simulink model "pendule_simple"  (R2016a)
settings: Solver=VariableStepAuto  StartTime=0.0  StopTime=10.0  RelTol=1e-3
undefined symbols (not defined in the file): K
libraries: simulink x1
settings Model: Creator=tmeunier  LastModifiedBy=tmeunier

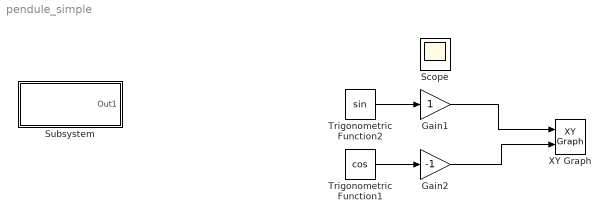
== system pendule_simple ==
  Gain1 : Gain
  Gain2 : Gain  Gain=-1
  Scope : Scope
  Subsystem : Subsystem
  Trigonometric Function1 : Trigonometry  Operator=cos
  Trigonometric Function2 : Trigonometry
  XY Graph : simulink/Sinks/XY Graph  xmin=-1  xmax=1  ymin=-1  ymax=1  st=-1
  wires:
  Gain1/1 -> XY Graph/1
  Trigonometric Function2/1 -> Gain1/1
  Trigonometric Function1/1 -> Gain2/1
  Gain2/1 -> XY Graph/2

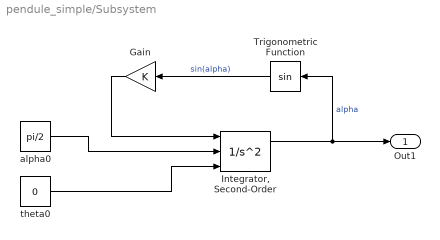
== system pendule_simple/Subsystem ==
  Gain : Gain  Gain=K
  "Integrator, Second-Order" : SecondOrderIntegrator  ICSourceX=external  ICSourceDXDT=external
  Trigonometric Function : Trigonometry
  alpha0 : Constant  Value=pi/2
  theta0 : Constant  Value=0
  Out1 : Outport
  wires:
  Trigonometric Function/1 -> Gain/1  "sin(alpha)"
  theta0/1 -> "Integrator, Second-Order"/3
  Gain/1 -> "Integrator, Second-Order"/1
  alpha0/1 -> "Integrator, Second-Order"/2
  "Integrator, Second-Order"/1 -> Out1/1, Trigonometric Function/1  "alpha"
